simulink model "smallsailboat"  (R2022b)
settings: Solver=VariableStepAuto  StartTime=0.0  StopTime=15  RelTol=1e-3
settings Model: Creator=ruben  LastModifiedBy=ruben

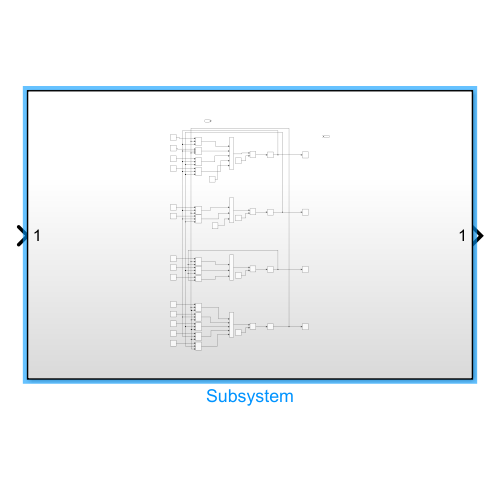
[thumbnail: Simulink's stored preview of the top-level diagram]
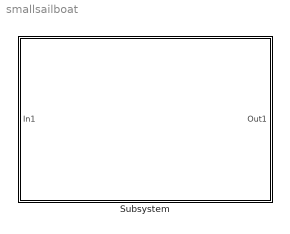
== system smallsailboat ==
  Subsystem : Subsystem

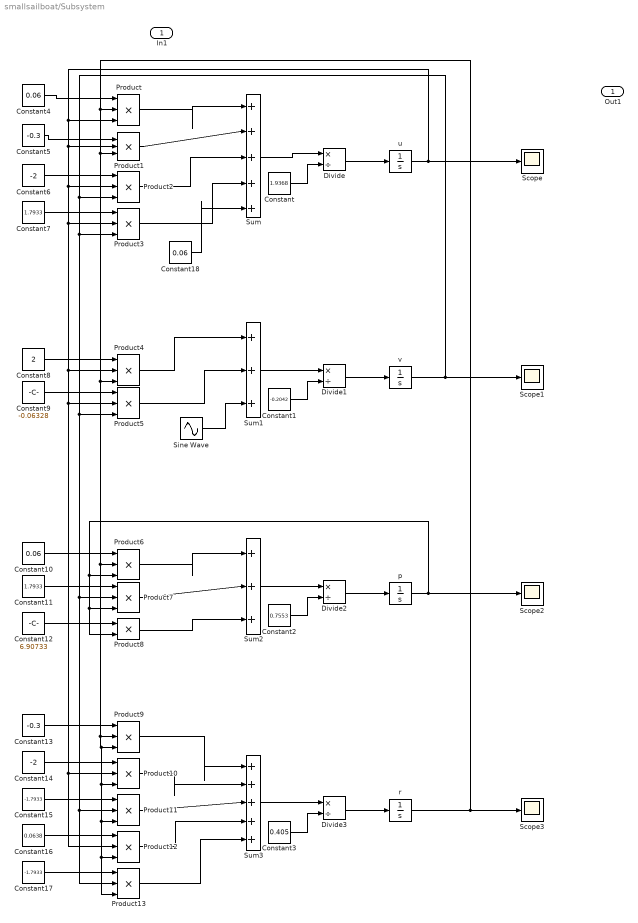
== system smallsailboat/Subsystem ==
  In1 : Inport
  Constant : Constant  Value=1.9368
  Constant1 : Constant  Value=-0.2042
  Constant10 : Constant  Value=0.06
  Constant11 : Constant  Value=1.7933
  Constant12 : Constant  Value=6.90733
  Constant13 : Constant  Value=-0.3
  Constant14 : Constant  Value=-2
  Constant15 : Constant  Value=-1.7933
  Constant16 : Constant  Value=0.0638
  Constant17 : Constant  Value=-1.7933
  Constant18 : Constant  Value=0.06
  Constant2 : Constant  Value=0.7553
  Constant3 : Constant  Value=0.405
  Constant4 : Constant  Value=0.06
  Constant5 : Constant  Value=-0.3
  Constant6 : Constant  Value=-2
  Constant7 : Constant  Value=1.7933
  Constant8 : Constant  Value=2
  Constant9 : Constant  Value=-0.06328
  Divide{,1..3} (4 alike) : Product  Inputs=*/
  Product{,1..7,9..13} (13 alike) : Product  Inputs=3
  Product8 : Product
  Scope{,1..3} (4 alike) : Scope
  Sine Wave : Sin  Amplitude=0.01  SampleTime=0
  Sum : Sum  Inputs=|+++++
  Sum1 : Sum  Inputs=|+++
  Sum2 : Sum  Inputs=|+++
  Sum3 : Sum  Inputs=|+++++
  p : Integrator
  r : Integrator
  u : Integrator
  v : Integrator
  Out1 : Outport
  wires:
  Sum/1 -> Divide/1
  Divide/1 -> u/1
  Constant/1 -> Divide/2
  Constant1/1 -> Divide1/2
  Sum1/1 -> Divide1/1
  Divide1/1 -> v/1
  Constant2/1 -> Divide2/2
  Sum2/1 -> Divide2/1
  Divide2/1 -> p/1
  Constant3/1 -> Divide3/2
  Sum3/1 -> Divide3/1
  Divide3/1 -> r/1
  Product/1 -> Sum/1
  Constant4/1 -> Product/1
  r/1 -> Scope3/1, Product13/3, Product12/3, Product11/3, Product10/3, Product9/3, Product9/2, Product6/2, Product4/3, Product1/3, Product/2
  u/1 -> Scope/1, Product/3, Product1/2, Product12/2, Product10/2, Product5/2, Product4/2, Product3/2, Product2/2
  Product1/1 -> Sum/2
  Product2/1 -> Sum/3
  Product3/1 -> Sum/4
  Constant5/1 -> Product1/1
  Constant6/1 -> Product2/1
  v/1 -> Scope1/1, Product13/2, Product11/2, Product7/2, Product5/3, Product3/3, Product2/3
  Constant7/1 -> Product3/1
  Product4/1 -> Sum1/1
  Product5/1 -> Sum1/2
  Constant8/1 -> Product4/1
  Constant9/1 -> Product5/1
  Product6/1 -> Sum2/1
  Product7/1 -> Sum2/2
  Product8/1 -> Sum2/3
  Constant10/1 -> Product6/1
  Constant11/1 -> Product7/1
  Constant12/1 -> Product8/1
  Product9/1 -> Sum3/1
  Product10/1 -> Sum3/2
  Product11/1 -> Sum3/3
  Product12/1 -> Sum3/4
  Product13/1 -> Sum3/5
  Constant13/1 -> Product9/1
  Constant14/1 -> Product10/1
  Constant15/1 -> Product11/1
  Constant16/1 -> Product12/1
  Constant17/1 -> Product13/1
  p/1 -> Scope2/1, Product8/2, Product7/3, Product6/3
  Constant18/1 -> Sum/5
  Sine Wave/1 -> Sum1/3
